simulink model "simulink_w1"  (R2025a)
settings: Solver=VariableStepAuto  StartTime=0.0  StopTime=450  RelTol=1e-3
undefined symbols (not defined in the file or in its folder): carData
settings Model: Creator=luke_  LastModifiedBy=luke_

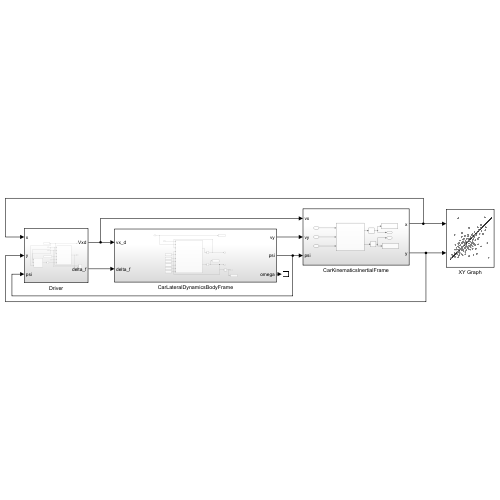
[thumbnail: Simulink's stored preview of the top-level diagram]
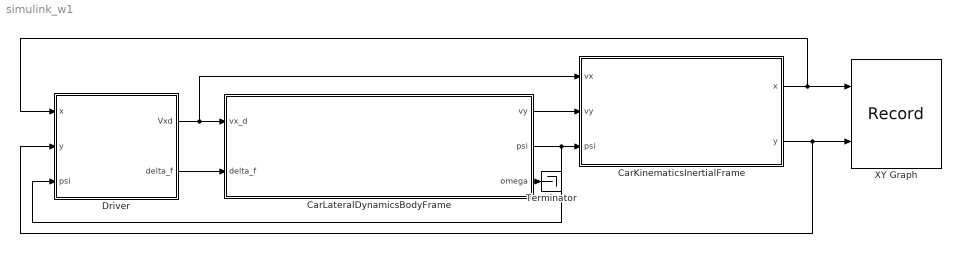
== system simulink_w1 ==
  CarKinematicsInertialFrame : Subsystem
  CarLateralDynamicsBodyFrame : Subsystem
  Driver : Subsystem
  Terminator : Terminator
  XY Graph : Record  NumPorts=2.0  FileSettingsInternal="{\"entries\":[{\"content\":{\"excelSettings\":{\"content\":{},\"type\":\"Streamout.ExcelSettings\"},\"parquetSettings\":{\"content\":{},\"type\":\"Streamout.ParquetSettings\"}},\"type\":\"Streamout.FileSettingStorage\",\"uuid\":\"\"}],\"packageUris\":[\"http:\\/\\/schema.mathworks.com\\/mf0\\/streamout_blocks\\/R2020a\"],\"version\":\"1.0\"}"  FrameSettings=[0, 0]  Layout=[1 1]  SignalsInternal="{\"entries\":[{\"content\":{\"signals\":[{\"content\":{\"blockPath\":[],\"dimensions\":[1],\"domain\":\"\",\"lineColor\":\"#a2142f\",\"plots\":[ 1 ],\"port\":1,\"sid\":[\"\"],\"signalID\":1,\"signalName\":\"CarKinematicsInertialFrame:1\"},\"type\":\"RecordBlkView.Signal\",\"uuid\":\"\"},{\"content\":{\"blockPath\":[],\"dimensions\":[1],\"domain\":\"\",\"lineColor\":\"#139fff\",\"plots\":[ 1 ],\"port\":2,\"sid\":[\"\"],\"signalID\":2,\"signalName\":\"CarKinematicsInertialFrame:2\"},\"type\":\"RecordBlkView.Signal\",\"uuid\":\"\"}]},\"type\":\"RecordBlkView.InputSignals\",\"uuid\":\"\"}],\"packageUris\":[\"http:\\/\\/schema.mathworks.com\\/mf0\\/streamout_blocks\\/R2020a\"],\"version\":\"1.0\"}"  VisualizationBindings="{\"xyplotplugin\":{\"info\":[{\"series\":[{\"bindingParametersList\":[{\"parameter\":\"X-Axis\",\"signalID\":1,\"signalName\":\"CarKinematicsInertialFrame:1\"},{\"parameter\":\"Y-Axis\",\"signalID\":2,\"signalName\":\"CarKinematicsInertialFrame:2\"}],\"seriesID\":0}],\"subplotID\":1}]}}"  CompatibilityTag=XY
  wires:
  Driver/2(delta_f) -> CarLateralDynamicsBodyFrame/2(delta_f)
  Driver/1(Vxd) -> CarLateralDynamicsBodyFrame/1(vx_d), CarKinematicsInertialFrame/1(vx)
  CarLateralDynamicsBodyFrame/1(vy) -> CarKinematicsInertialFrame/2(vy)
  CarLateralDynamicsBodyFrame/2(psi) -> Driver/3(psi), CarKinematicsInertialFrame/3(psi)
  CarKinematicsInertialFrame/1(x) -> Driver/1(x), XY Graph/1
  CarKinematicsInertialFrame/2(y) -> Driver/2(y), XY Graph/2
  CarLateralDynamicsBodyFrame/3(omega) -> Terminator/1

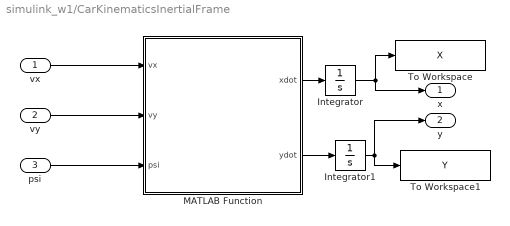
== system simulink_w1/CarKinematicsInertialFrame ==
  vx : Inport
  vy : Inport  Port=2
  psi : Inport  Port=3
  Integrator : Integrator  InitialCondition=carData.init.X0
  Integrator1 : Integrator  InitialCondition=carData.init.Y0
  MATLAB Function : MATLAB Function  TreatAsAtomicUnit=on
  To Workspace : ToWorkspace  VariableName=X  SaveFormat=Timeseries  SampleTime=-1
  To Workspace1 : ToWorkspace  VariableName=Y  SaveFormat=Timeseries  SampleTime=-1
  x : Outport
  y : Outport  Port=2
  wires:
  vx/1 -> MATLAB Function/1(vx)
  vy/1 -> MATLAB Function/2(vy)
  psi/1 -> MATLAB Function/3(psi)
  MATLAB Function/1(xdot) -> Integrator/1
  MATLAB Function/2(ydot) -> Integrator1/1
  Integrator/1 -> To Workspace/1, x/1
  Integrator1/1 -> To Workspace1/1, y/1

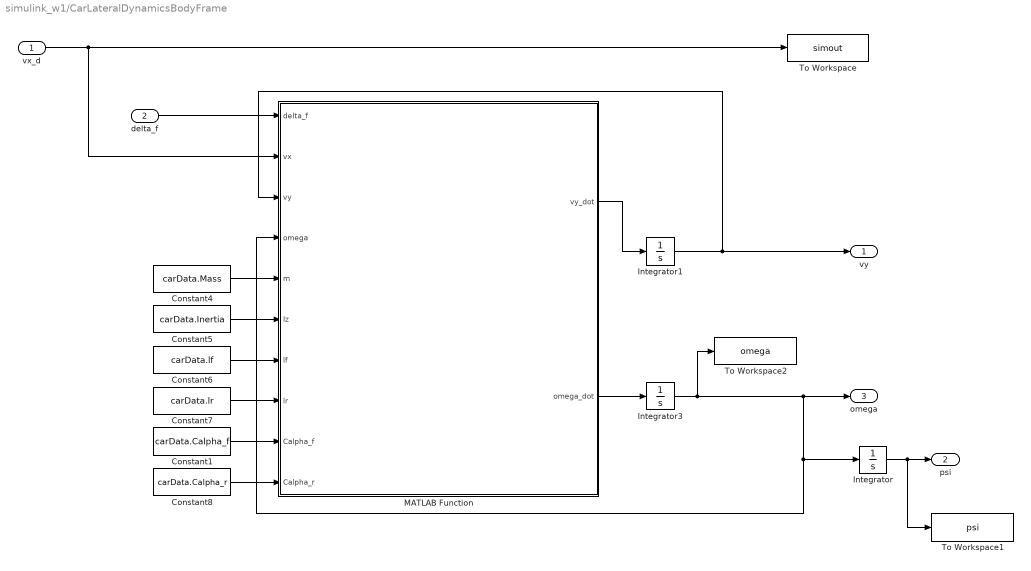
== system simulink_w1/CarLateralDynamicsBodyFrame ==
  vx_d : Inport
  delta_f : Inport  Port=2
  Constant1 : Constant  Value=carData.Calpha_f
  Constant4 : Constant  Value=carData.Mass
  Constant5 : Constant  Value=carData.Inertia
  Constant6 : Constant  Value=carData.lf
  Constant7 : Constant  Value=carData.lr
  Constant8 : Constant  Value=carData.Calpha_r
  Integrator : Integrator
  Integrator1 : Integrator
  Integrator3 : Integrator
  MATLAB Function : MATLAB Function  TreatAsAtomicUnit=on
  To Workspace : ToWorkspace  VariableName=simout  SaveFormat=Timeseries  SampleTime=-1
  To Workspace1 : ToWorkspace  VariableName=psi  SaveFormat=Timeseries  SampleTime=-1
  To Workspace2 : ToWorkspace  VariableName=omega  SaveFormat=Timeseries  SampleTime=-1
  vy : Outport
  psi : Outport  Port=2
  omega : Outport  Port=3
  wires:
  vx_d/1 -> To Workspace/1, MATLAB Function/2(vx)
  delta_f/1 -> MATLAB Function/1(delta_f)
  Constant4/1 -> MATLAB Function/5(m)
  Constant5/1 -> MATLAB Function/6(Iz)
  Constant6/1 -> MATLAB Function/7(lf)
  Constant7/1 -> MATLAB Function/8(lr)
  Constant1/1 -> MATLAB Function/9(Calpha_f)
  Constant8/1 -> MATLAB Function/10(Calpha_r)
  MATLAB Function/1(vy_dot) -> Integrator1/1
  Integrator1/1 -> MATLAB Function/3(vy), vy/1
  MATLAB Function/2(omega_dot) -> Integrator3/1
  Integrator3/1 -> MATLAB Function/4(omega), Integrator/1, omega/1, To Workspace2/1
  Integrator/1 -> psi/1, To Workspace1/1

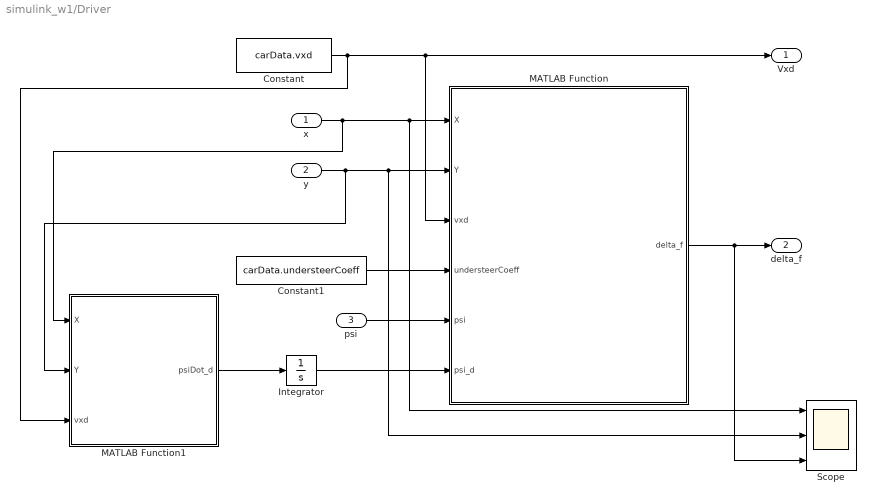
== system simulink_w1/Driver ==
  x : Inport
  y : Inport  Port=2
  psi : Inport  Port=3
  Constant : Constant  Value=carData.vxd
  Constant1 : Constant  Value=carData.understeerCoeff
  Integrator : Integrator
  MATLAB Function : MATLAB Function  TreatAsAtomicUnit=on
  MATLAB Function1 : MATLAB Function  TreatAsAtomicUnit=on
  Scope : Scope  NumInputPorts=3
  Vxd : Outport
  delta_f : Outport  Port=2
  wires:
  x/1 -> MATLAB Function1/1(X), Scope/1, MATLAB Function/1(X)
  y/1 -> MATLAB Function1/2(Y), Scope/2, MATLAB Function/2(Y)
  Constant/1 -> MATLAB Function1/3(vxd), MATLAB Function/3(vxd), Vxd/1
  MATLAB Function/1(delta_f) -> delta_f/1, Scope/3
  psi/1 -> MATLAB Function/5(psi)
  Constant1/1 -> MATLAB Function/4(understeerCoeff)
  MATLAB Function1/1(psiDot_d) -> Integrator/1
  Integrator/1 -> MATLAB Function/6(psi_d)

== matlab function simulink_w1/Driver/MATLAB Function ==
  data: X input; delta_f output; Y input; vxd input; understeerCoeff input; psi input; psi_d input
function delta_f = Driver(X, Y, vxd, understeerCoeff, psi, psi_d)

% function delta_f = Driver(X, Y, vxd, understeerCoeff, psi)
    R = 200;       % radius of the turn
    Ls = 900;      % length of straightaway
    eps = 1e-9;
    L = 2.5;       % wheelbase
    Kp = 0.085;      % proportional gain for heading error, was 0.075

    e = psi_d - psi;       % heading error
    ack = L / R;           % feedforward Ackermann angle
    damping = understeerCoeff * vxd^2;  % understeer correction

    % Default: no steering
    delta_f = 0;

    % If outside the straightaway, apply feedback + feedforward
    if (X < 0 -eps) || (X > Ls + eps)
        delta_f = Kp * e + ack + damping;

    % On straightaway, apply small corrections based on lateral position
    elseif X > 0 && X < Ls && Y > 401
        delta_f = 0.0015;

    elseif X > 0 && X < Ls && Y < 400 && Y > 390
        delta_f = -0.0015;
    %on bottom straightaway
    elseif X > 0 && X < Ls && Y < -5
        delta_f = 0.0015;

    elseif X > 0 && X < Ls && Y > 5
        delta_f = -0.0015;

    end
end

== matlab function simulink_w1/CarKinematicsInertialFrame/MATLAB Function ==
  data: vx input; xdot output; vy input; psi input; ydot output
function [xdot, ydot] = fcn(vx, vy, psi)
    % Transform body-frame velocity to global frame
    temp = TF(psi) * [vx; vy];
    xdot = temp(1);
    ydot = temp(2);


end

function y = TF(psi)
    y = [cos(psi), -sin(psi); sin(psi), cos(psi)];
end

== matlab function simulink_w1/CarLateralDynamicsBodyFrame/MATLAB Function ==
  data: delta_f input; vx input; vy input; omega input; m input; Iz input; lf input; lr input; Calpha_f input; Calpha_r input; vy_dot output; omega_dot output
function [vy_dot, omega_dot] = lateralDynamics(delta_f, vx, vy, omega, m, Iz, lf, lr, Calpha_f, Calpha_r)
% Implements linearized lateral dynamics model with small angle assumption

% Avoid division by zero
vx = max(vx, 0.1);

% Compute lateral tire forces (linear tire model)
Fyf = -Calpha_f * (-delta_f - (vy + lf * omega) / vx);
Fyr = -Calpha_r * ((vy - lr * omega) / vx);

% Lateral acceleration
vy_dot = (Fyf + Fyr) / m - omega * vx;

% Yaw acceleration
omega_dot = (lf * Fyf - lr * Fyr) / Iz;
end

== matlab function simulink_w1/Driver/MATLAB Function1 ==
  data: X input; psiDot_d output; Y input; vxd input
function psiDot_d = DediredHeadingRate(X, Y, vxd)

R = 200;
Ls = 900;
eps = 1e-9;
    if (X <0 -eps) || (X > Ls + eps) %if outside straightaway
        psiDot_d = vxd/R;

    else                            % inside the turns 
        psiDot_d = 0;


    end 

 end
